simulink model "linear_quad"  (R2015b)
settings: Solver=VariableStepAuto  StartTime=0.0  StopTime=50  RelTol=1e-3
libraries: simulink x4
settings Model: Creator=zachn  LastModifiedBy=reldn_000
settings ConfigComp: CovModelRefEnable=Off

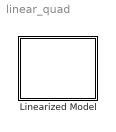
== system linear_quad ==
  Linearized Model : Subsystem  mask{m=0.468, Ixyz=[4.856e-3 4.856e-3 8.801e-3], r=0.225, Kl=2.980e-6, Kb=1.140e-7, zdt_cmd=0, r_cmd=.5*pi/180, p_cmd=0*pi/180, ydt_cmd=0*pi/180}
      mask prompts: m "Mass (kg)"; Ixyz "Inertia, Ixyz (kg m^2)"; r "Arm Radius (m)"; Kl "Lift Constant"; Kb "Drag Constant"; zdt_cmd "Z velocity [m/s] (positive down)"; r_cmd "Roll angle [rad]"; p_cmd "Pitch angle [rad]"; ydt_cmd "Yaw rate [rad/s]"
      mask init:
      | % define the inertia matrix, I, from the given components
      | I = [   Ixyz(1)     0       0   ;...
      |             0   Ixyz(2)     0   ;...
      |             0       0   Ixyz(3) ; ...
      |     ];
      | 
      | hover_offset = sqrt((m*9.81)/(4*Kl));

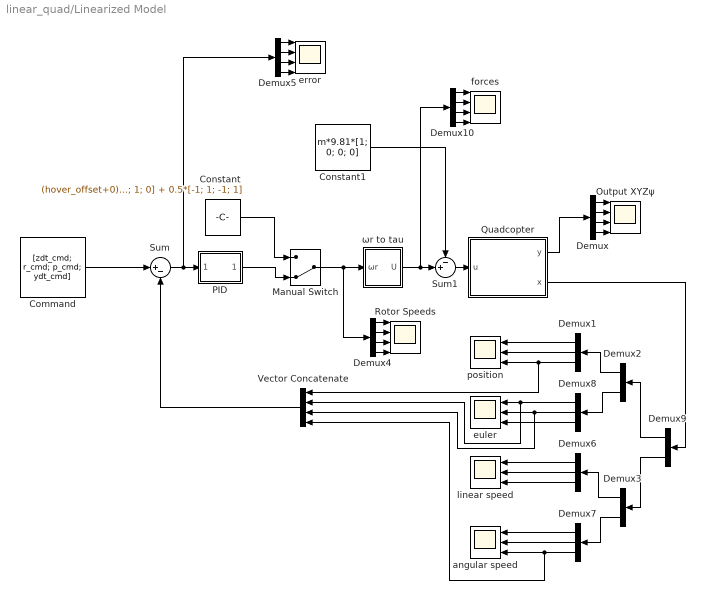
== system linear_quad/Linearized Model ==
  Command : Constant  Value=[zdt_cmd; r_cmd; p_cmd; ydt_cmd]  VectorParams1D=off
  Constant : Constant  Value="(hover_offset+0)*[1; 1; 1; 1] + 0*[0; -1; 0; 1]  + 0*[-1; 0; 1; 0] + 0.5*[-1; 1; -1; 1]"  VectorParams1D=off
  Constant1 : Constant  Value=m*9.81*[1; 0; 0; 0]  VectorParams1D=off
  Demux{,4..5,10} (4 alike) : Demux
  Demux{1,6..8} (4 alike) : Demux  Outputs=3
  Demux2 : Demux  Outputs=2
  Demux3 : Demux  Outputs=2
  Demux9 : Demux  Outputs=2
  Manual Switch : ManualSwitch  CurrentSetting=0
  Output XYZψ : Scope  NumInputPorts=4
  PID : Subsystem  mask{zdt_P=1, zdt_I=0, zdt_D=0, roll_P=1, roll_I=0, roll_D=0, pitch_P=1, pitch_I=0, pitch_D=0, yaw_rate_P=1, yaw_rate_I=0, yaw_rate_D=0}
      mask prompts: zdt_P "P"; zdt_I "I"; zdt_D "D"; roll_P "P"; roll_I "I"; roll_D "D"; pitch_P "P"; pitch_I "I"; pitch_D "D"; yaw_rate_P "P"; yaw_rate_I "I"; yaw_rate_D "D"
  Quadcopter : Subsystem  mask{m=m, i_xyz=I, g=9.81, A=0, B=0, C=0, D=0}
      mask prompts: m "Mass (kg)"; i_xyz "Moment of Inertia Ixyz (kg m^2)"; g "Gravity (m/s^2)"; A "A Matrix"; B "B Matrix"; C "C Matrix"; D "D Matrix"
      mask init:
      | % state space model based off IEEE paper by Araar and Aouf, which
      | % linearizes the model by assuming an equilibrium point at hovering.
      | % The state maxtrix x is as follows:
      | % x = [x y z roll pitch yaw x_dt y_dt z_dt roll_dt pitch_dt yaw_dt]
      | % y = [x y z yaw]
      | %
      | % This uses the following assumptions:
      | % thrust = mg
      | % linear speeds w.r.t the body frame are all 0
      | % sin(yaw) = 0 -> means pitch controls x position and roll controls y, both
      | % w.r.t the inertial (earth) frame
      | % sin(theta) = theta (pitch)
      | % sin(phi) = phi (roll)
      | 
      | A = [
      |         zeros(3,4)  zeros(3,1)  zeros(3,1)  i_xyz       zeros(3,3)  ; ...
      |         zeros(3,4)  zeros(3,1)  zeros(3,1)  zeros(3,3)  i_xyz       ; ...
      |         zeros(1,4)  zeros(1,1)      g       zeros(1,3)  zeros(1,3)  ; ...
      |         zeros(1,4)      -g      zeros(1,1)  zeros(1,3)  zeros(1,3)  ; ...
      |         zeros(4,4)  zeros(4,1)  zeros(4,1)  zeros(4,3)  zeros(4,3)    ...
      |     ];
      | 
      | B = [
      |         zeros(8,1)  zeros(8,1)  zeros(8,1)  zeros(8,1)  ; ...
      |             1/m         0           0           0       ; ...
      |             0       1/i_xyz(1,1)    0           0       ; ...
      |             0           0       1/i_xyz(2,2)    0       ; ...
      |             0           0           0       1/i_xyz(3,3)  ...
      |     ];
      | 
      | C = [
      |         i_xyz       zeros(3,2)  zeros(3,1)  zeros(3,6)  ; ...
      |         zeros(1,3)  zeros(1,2)      1       zeros(1,6)    ...
      |     ];
      | 
      | D = zeros(4,4); % null matrix
      | 
      | % A = [   zeros(3,3), eye(3,3), zeros(3,6)    ; ...
      | %         zeros(3,12)                         ; ...
      | %         0, -g, zeros(1,10)                  ; ...
      | %         g, zeros(1,11)                      ; ...
      | %         zeros(1,12)                         ; ...
      | %         zeros(3,6), eye(3,3), zeros(3,3)      ...
      | %     ];
      | % 
      | % B = [   zeros(3,4)              ; ...
      | %         0, 1/i_xyz(1), 0, 0     ; ...
      | %         0, 0, 1/i_xyz(2), 0     ; ...
      | %         0, 0, 0, 1/i_xyz(3)     ; ...
      | %         zeros(2,4)              ; ...
      | %         1/m, 0, 0, 0            ; ...
      | %         0,   0, 0, 0              ...
      | %     ];
      | % 
      | % C = [   zeros(1,9),     1, zeros(1,2)   ; ...
      | %         zeros(1,10),    1, zeros(1,1)   ; ...
      | %         zeros(1,11),    1               ; ...
      | %         zeros(1,2),     1, zeros(1,9)     ...
      | %      ];
      |  
      | %  D = [  zeros(3,6)                  ; ...
      | %         zeros(1,3) 1/i_xyz(1) 0 0   ; ...
      | %         zeros(1,4) 1/i_xyz(2) 0     ; ...
      | %         zeros(1,5) 1/i_xyz(3)       ; ...
      | %         1/m 0 0 0 0 0               ; ...
      | %         0 1/m 0 0 0 0               ; ...
      | %         0 0 1/m 0 0 0               ; ...
      | %         0 0 0 1/m 0 0               ; ...
      | %         zeros(3,6)                    ...
      | %      ];
      mask DialogControl DescGroupVar Prompt: Linearized State Space Model
      mask DialogControl DescTextVar Prompt: Dynamic model of a quadcopter represented in state space form. Model is linearized around a hovering state at which the system is in equilibrium. This uses the assumptions that thrust is roughly equivalent to gravity and that the yaw angle is 0.
      mask DialogControl Control2 Prompt: GET TO THE QUADCOPTA!!!
      mask DialogControl Control2 Callback: web www.youtube.com/watch?v=Xs_OacEq2Sk
      mask DialogControl Container4 Prompt: System Parameters
  Rotor Speeds : Scope  NumInputPorts=4
  Sum : Sum  Inputs=|+-
  Sum1 : Sum  Inputs=-+|
  Vector Concatenate : Concatenate  NumInputs=4  Mode=Multidimensional array
  angular speed : Scope  NumInputPorts=3
  error : Scope  NumInputPorts=4
  euler : Scope  NumInputPorts=3
  forces : Scope  NumInputPorts=4
  linear speed : Scope  NumInputPorts=3
  position : Scope  NumInputPorts=3
  ωr to tau : Subsystem
  wires:
  Demux/1 -> Output XYZψ/1
  Demux/2 -> Output XYZψ/2
  Demux/3 -> Output XYZψ/3
  Demux/4 -> Output XYZψ/4
  Quadcopter/1(y) -> Demux/1
  Demux8/1 -> Vector Concatenate/2, euler/1
  Demux8/3 -> euler/3
  Demux7/3 -> Vector Concatenate/4, angular speed/3
  Demux8/2 -> Vector Concatenate/3, euler/2
  Demux7/2 -> angular speed/2
  Demux3/1 -> Demux6/1
  Demux3/2 -> Demux7/1
  Demux6/1 -> linear speed/1
  Demux6/2 -> linear speed/2
  Demux6/3 -> linear speed/3
  Demux7/1 -> angular speed/1
  Quadcopter/2(x) -> Demux9/1
  Demux9/2 -> Demux3/1
  Demux1/2 -> position/2
  Demux1/1 -> position/1
  Demux2/1 -> Demux1/1
  Demux2/2 -> Demux8/1
  Demux9/1 -> Demux2/1
  Vector Concatenate/1 -> Sum/2
  Demux1/3 -> Vector Concatenate/1, position/3
  Command/1 -> Sum/1
  PID/1(ω r) -> Manual Switch/2
  Constant/1 -> Manual Switch/1
  Demux5/2 -> error/2
  Demux5/4 -> error/4
  Demux5/3 -> error/3
  Demux5/1 -> error/1
  Sum/1 -> Demux5/1, PID/1(cmd)
  Sum1/1 -> Quadcopter/1(u)
  Demux4/1 -> Rotor Speeds/1
  Demux4/3 -> Rotor Speeds/3
  Demux4/2 -> Rotor Speeds/2
  Demux4/4 -> Rotor Speeds/4
  Demux10/1 -> forces/1
  Demux10/3 -> forces/3
  Demux10/4 -> forces/4
  Demux10/2 -> forces/2
  ωr to tau/1(U) -> Demux10/1, Sum1/2
  Constant1/1 -> Sum1/1
  Manual Switch/1 -> Demux4/1, ωr to tau/1(ωr)

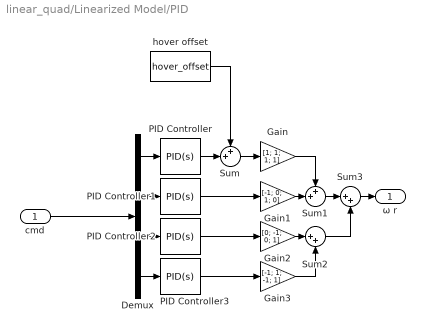
== system linear_quad/Linearized Model/PID ==
  cmd : Inport
  Demux : Demux
  Gain : Gain  Gain=[1; 1; 1; 1]
  Gain1 : Gain  Gain=[-1; 0; 1; 0]
  Gain2 : Gain  Gain=[0; -1; 0; 1]
  Gain3 : Gain  Gain=[-1; 1; -1; 1]
  PID Controller : simulink/Continuous/PID Controller  Controller=PID  Form=Parallel  TimeDomain=Continuous-time  SampleTime=-1  IntegratorMethod=Forward Euler  FilterMethod=Forward Euler  ControllerParametersSource=internal  P=zdt_P  I=zdt_I  D=zdt_D  UseFilter=on  N=3.695  InitialConditionSource=internal  InitialConditionForIntegrator=0  InitialConditionForFilter=0  DifferentiatorICPrevScaledInput=0  ExternalReset=none  TrackingMode=off  Kt=1  LimitOutput=off  UpperSaturationLimit=inf  LowerSaturationLimit=-inf  LinearizeAsGain=on  AntiWindupMode=none  Kb=1  POutMin=[]  POutMax=[]  IOutMin=[]  IOutMax=[]  DOutMin=[]  DOutMax=[]  NOutMin=[]  NOutMax=[]  SumOutMin=[]  SumOutMax=[]  SaturationOutMin=[]  SaturationOutMax=[]  PParamMin=[]  PParamMax=[]  IParamMin=[]  IParamMax=[]  DParamMin=[]  DParamMax=[]  NParamMin=[]  NParamMax=[]  KbParamMin=[]  KbParamMax=[]  KtParamMin=[]  KtParamMax=[]  KbOutMin=[]  KbOutMax=[]  KtOutMin=[]  KtOutMax=[]  IntegratorOutMin=[]  IntegratorOutMax=[]  FilterOutMin=[]  FilterOutMax=[]  SumI1OutMin=[]  SumI1OutMax=[]  SumI2OutMin=[]  SumI2OutMax=[]  SumI3OutMin=[]  SumI3OutMax=[]  SumDOutMin=[]  SumDOutMax=[]  DifferentiatorOutMin=[]  DifferentiatorOutMax=[]  IntegratorContinuousStateAttributes=''  IntegratorStateMustResolveToSignalObject=off  IntegratorRTWStateStorageClass=Auto  FilterContinuousStateAttributes=''  FilterStateMustResolveToSignalObject=off  FilterRTWStateStorageClass=Auto
  PID Controller1 : simulink/Continuous/PID Controller  Controller=PID  Form=Parallel  TimeDomain=Continuous-time  SampleTime=-1  IntegratorMethod=Forward Euler  FilterMethod=Forward Euler  ControllerParametersSource=internal  P=roll_P  I=roll_I  D=roll_D  UseFilter=on  N=114.3  InitialConditionSource=internal  InitialConditionForIntegrator=0  InitialConditionForFilter=0  DifferentiatorICPrevScaledInput=0  ExternalReset=none  TrackingMode=off  Kt=1  LimitOutput=off  UpperSaturationLimit=inf  LowerSaturationLimit=-inf  LinearizeAsGain=on  AntiWindupMode=none  Kb=1  POutMin=[]  POutMax=[]  IOutMin=[]  IOutMax=[]  DOutMin=[]  DOutMax=[]  NOutMin=[]  NOutMax=[]  SumOutMin=[]  SumOutMax=[]  SaturationOutMin=[]  SaturationOutMax=[]  PParamMin=[]  PParamMax=[]  IParamMin=[]  IParamMax=[]  DParamMin=[]  DParamMax=[]  NParamMin=[]  NParamMax=[]  KbParamMin=[]  KbParamMax=[]  KtParamMin=[]  KtParamMax=[]  KbOutMin=[]  KbOutMax=[]  KtOutMin=[]  KtOutMax=[]  IntegratorOutMin=[]  IntegratorOutMax=[]  FilterOutMin=[]  FilterOutMax=[]  SumI1OutMin=[]  SumI1OutMax=[]  SumI2OutMin=[]  SumI2OutMax=[]  SumI3OutMin=[]  SumI3OutMax=[]  SumDOutMin=[]  SumDOutMax=[]  DifferentiatorOutMin=[]  DifferentiatorOutMax=[]  IntegratorContinuousStateAttributes=''  IntegratorStateMustResolveToSignalObject=off  IntegratorRTWStateStorageClass=Auto  FilterContinuousStateAttributes=''  FilterStateMustResolveToSignalObject=off  FilterRTWStateStorageClass=Auto
  PID Controller2 : simulink/Continuous/PID Controller  Controller=PID  Form=Parallel  TimeDomain=Continuous-time  SampleTime=-1  IntegratorMethod=Forward Euler  FilterMethod=Forward Euler  ControllerParametersSource=internal  P=pitch_P  I=pitch_I  D=pitch_D  UseFilter=on  N=114.3  InitialConditionSource=internal  InitialConditionForIntegrator=0  InitialConditionForFilter=0  DifferentiatorICPrevScaledInput=0  ExternalReset=none  TrackingMode=off  Kt=1  LimitOutput=off  UpperSaturationLimit=inf  LowerSaturationLimit=-inf  LinearizeAsGain=on  AntiWindupMode=none  Kb=1  POutMin=[]  POutMax=[]  IOutMin=[]  IOutMax=[]  DOutMin=[]  DOutMax=[]  NOutMin=[]  NOutMax=[]  SumOutMin=[]  SumOutMax=[]  SaturationOutMin=[]  SaturationOutMax=[]  PParamMin=[]  PParamMax=[]  IParamMin=[]  IParamMax=[]  DParamMin=[]  DParamMax=[]  NParamMin=[]  NParamMax=[]  KbParamMin=[]  KbParamMax=[]  KtParamMin=[]  KtParamMax=[]  KbOutMin=[]  KbOutMax=[]  KtOutMin=[]  KtOutMax=[]  IntegratorOutMin=[]  IntegratorOutMax=[]  FilterOutMin=[]  FilterOutMax=[]  SumI1OutMin=[]  SumI1OutMax=[]  SumI2OutMin=[]  SumI2OutMax=[]  SumI3OutMin=[]  SumI3OutMax=[]  SumDOutMin=[]  SumDOutMax=[]  DifferentiatorOutMin=[]  DifferentiatorOutMax=[]  IntegratorContinuousStateAttributes=''  IntegratorStateMustResolveToSignalObject=off  IntegratorRTWStateStorageClass=Auto  FilterContinuousStateAttributes=''  FilterStateMustResolveToSignalObject=off  FilterRTWStateStorageClass=Auto
  PID Controller3 : simulink/Continuous/PID Controller  Controller=PID  Form=Parallel  TimeDomain=Continuous-time  SampleTime=-1  IntegratorMethod=Forward Euler  FilterMethod=Forward Euler  ControllerParametersSource=internal  P=yaw_rate_P  I=yaw_rate_I  D=yaw_rate_D  UseFilter=on  N=3.647  InitialConditionSource=internal  InitialConditionForIntegrator=0  InitialConditionForFilter=0  DifferentiatorICPrevScaledInput=0  ExternalReset=none  TrackingMode=off  Kt=1  LimitOutput=off  UpperSaturationLimit=inf  LowerSaturationLimit=-inf  LinearizeAsGain=on  AntiWindupMode=none  Kb=1  POutMin=[]  POutMax=[]  IOutMin=[]  IOutMax=[]  DOutMin=[]  DOutMax=[]  NOutMin=[]  NOutMax=[]  SumOutMin=[]  SumOutMax=[]  SaturationOutMin=[]  SaturationOutMax=[]  PParamMin=[]  PParamMax=[]  IParamMin=[]  IParamMax=[]  DParamMin=[]  DParamMax=[]  NParamMin=[]  NParamMax=[]  KbParamMin=[]  KbParamMax=[]  KtParamMin=[]  KtParamMax=[]  KbOutMin=[]  KbOutMax=[]  KtOutMin=[]  KtOutMax=[]  IntegratorOutMin=[]  IntegratorOutMax=[]  FilterOutMin=[]  FilterOutMax=[]  SumI1OutMin=[]  SumI1OutMax=[]  SumI2OutMin=[]  SumI2OutMax=[]  SumI3OutMin=[]  SumI3OutMax=[]  SumDOutMin=[]  SumDOutMax=[]  DifferentiatorOutMin=[]  DifferentiatorOutMax=[]  IntegratorContinuousStateAttributes=''  IntegratorStateMustResolveToSignalObject=off  IntegratorRTWStateStorageClass=Auto  FilterContinuousStateAttributes=''  FilterStateMustResolveToSignalObject=off  FilterRTWStateStorageClass=Auto
  Sum : Sum  Inputs=++|
  Sum1 : Sum  Inputs=++|
  Sum2 : Sum  Inputs=|++
  Sum3 : Sum  Inputs=|++
  hover offset : Constant  Value=hover_offset
  ω r : Outport
  wires:
  cmd/1 -> Demux/1
  Demux/2 -> PID Controller1/1
  Demux/3 -> PID Controller2/1
  Demux/4 -> PID Controller3/1
  PID Controller1/1 -> Gain1/1
  PID Controller2/1 -> Gain2/1
  PID Controller3/1 -> Gain3/1
  Gain1/1 -> Sum1/2
  Gain2/1 -> Sum2/1
  Gain3/1 -> Sum2/2
  Sum1/1 -> Sum3/1
  Sum2/1 -> Sum3/2
  Sum3/1 -> ω r/1
  Gain/1 -> Sum1/1
  Demux/1 -> PID Controller/1
  hover offset/1 -> Sum/1
  PID Controller/1 -> Sum/2
  Sum/1 -> Gain/1

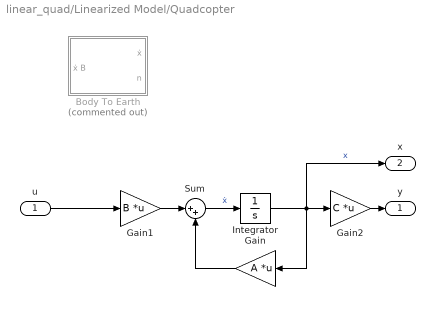
== system linear_quad/Linearized Model/Quadcopter ==
  u : Inport
  Body To Earth : Subsystem  Commented=on
  Gain : Gain  Gain=A  Multiplication=Matrix(K*u)
  Gain1 : Gain  Gain=B  Multiplication=Matrix(K*u)
  Gain2 : Gain  Gain=C  Multiplication=Matrix(K*u)
  Integrator : Integrator
  Sum : Sum  Inputs=|++
  y : Outport
  x : Outport  Port=2
  wires:
  Gain1/1 -> Sum/1
  Gain/1 -> Sum/2
  Sum/1 -> Integrator/1  "ẋ"
  Integrator/1 -> x/1, Gain2/1, Gain/1  "x"
  Gain2/1 -> y/1
  u/1 -> Gain1/1

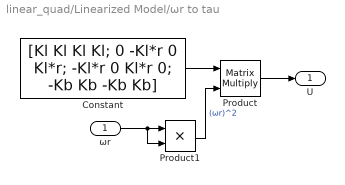
== system linear_quad/Linearized Model/ωr to tau ==
  ωr : Inport
  Constant : Constant  Value=[Kl Kl Kl Kl; 0 -Kl*r 0 Kl*r; -Kl*r 0 Kl*r 0; -Kb Kb -Kb Kb]  VectorParams1D=off
  Product : Product  Multiplication=Matrix(*)
  Product1 : Product
  U : Outport
  wires:
  Constant/1 -> Product/1
  Product/1 -> U/1
  ωr/1 -> Product1/2, Product1/1
  Product1/1 -> Product/2  "(ωr)^2"

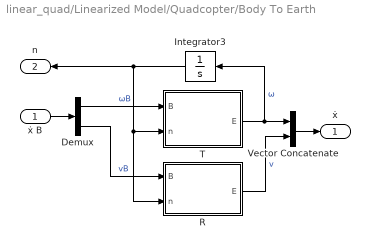
== system linear_quad/Linearized Model/Quadcopter/Body To Earth ==
  ẋ B : Inport
  Demux : Demux  Outputs=2
  Integrator3 : Integrator  InitialCondition=[0;0;0]
  R : MATLAB Function  TreatAsAtomicUnit=on
  T : MATLAB Function  TreatAsAtomicUnit=on
  Vector Concatenate : Concatenate  Mode=Multidimensional array
  ẋ : Outport
  n : Outport  Port=2
  wires:
  ẋ B/1 -> Demux/1
  Vector Concatenate/1 -> ẋ/1
  Integrator3/1 -> R/2(n), T/2(n), n/1
  T/1(E) -> Integrator3/1, Vector Concatenate/1  "ω"
  R/1(E) -> Vector Concatenate/2  "v"
  Demux/1 -> T/1(B)  "ωB"
  Demux/2 -> R/1(B)  "vB"

== matlab function linear_quad/Linearized Model/Quadcopter/Body To Earth/R ==
  data: B input size=[3;1]; E output; n input size=[3;1]
function E = body2earth(B,n)
% body2earth -  translates the given vector B expressed in the moving body
%               frame to the earth (stationary or inertial) frame.
%               
%               n is the vector containing the euler angles yaw, pitch, and
%               roll.

phi = n(1); % roll (phi)
the = n(2); % pitch (theta)
psi = n(3); % yaw (psi)

c_phi = cos(phi);
s_phi = sin(phi);
c_the = cos(the);
s_the = sin(the);
c_psi = cos(psi);
s_psi = sin(psi);

% The rotation matrix using the Euler transformation ZYX
Rzyx = [
c_the*c_psi, s_phi*s_the*c_psi-c_phi*s_psi, c_phi*s_the*c_psi+s_phi*s_psi ;...
c_the*s_psi, s_phi*s_the*s_psi+c_phi*c_psi, c_phi*s_the*s_psi-s_phi*c_psi ;...
-s_the       s_phi*c_the                    c_phi*c_the                   ;...
];

E = Rzyx*[B(1);B(2);B(3)];

== matlab function linear_quad/Linearized Model/Quadcopter/Body To Earth/T ==
  data: B input size=[3;1]; E output; n input size=[3;1]
function E = body2euler(B,n)
% body2euler -  Given the angular velocity vector of a moving body, B,
%               returns that vector expressed in the stationary (inertial)
%               frame of reference.
%
%               'n' is the vector containing euler angles roll, pitch, and
%               yaw

phi = n(1); % roll angle
the = n(2); % pitch angle

% angular transformation matrix. This is derived using the standard yaw,
% pitch, roll seqeuence.
T = [   1   sin(phi)*tan(the)   cos(phi)*tan(the)   ; ...
        0   cos(phi)            -sin(phi)           ; ...
        0   sin(phi)/cos(the)   cos(phi)/cos(the)   ; ...
    ];

E = T * [B(1);B(2);B(3)];
